simulink model "lab4_1"  (R2021b)
settings: Solver=VariableStepAuto  StartTime=0.0  StopTime=20.0  RelTol=10e-10  AbsTol=10e-10
values from neighbouring files (symbols this model uses):
  d_bar = (Ra/Kt)*tau_l    (= 3)    [lab4.m]
  thetades = pi/2    (= 1.57079632679)    [lab4.m]
  Vlim = 5    [lab4.m]
libraries: cstblocks x2
settings Model: Creator=jiayizhou  LastModifiedBy=jiayizhou

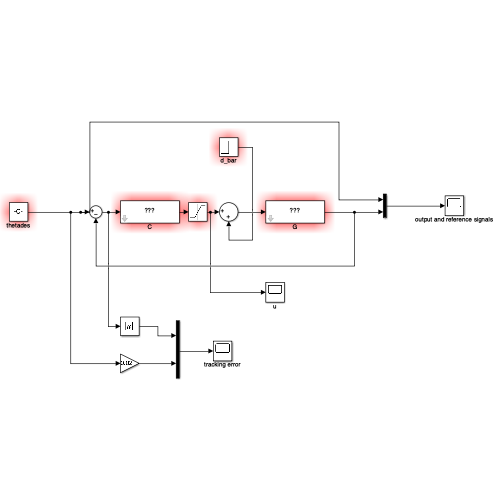
[thumbnail: Simulink's stored preview of the top-level diagram]
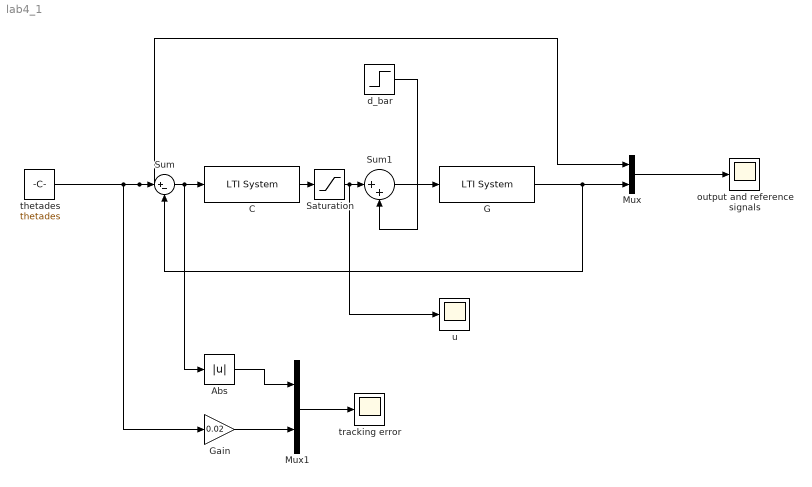
== system lab4_1 ==
  Abs : Abs
  C : cstblocks/LTI System  sys=C  IC=[]
  G : cstblocks/LTI System  sys=G  IC=[]
  Gain : Gain  Gain=0.02
  Mux : Mux  Inputs=2
  Mux1 : Mux  Inputs=2
  Saturation : Saturate  UpperLimit=Vlim  LowerLimit=-Vlim
  Sum : Sum  Inputs=|+-
  Sum1 : Sum  Inputs=|++
  d_bar : Step  Time=5  After=d_bar  SampleTime=0
  output and reference signals : Scope
  thetades : Constant  Value=thetades
  tracking error : Scope
  u : Scope
  wires:
  thetades/1 -> Gain/1, Mux/1, Sum/1
  Sum/1 -> Abs/1, C/1
  Sum1/1 -> G/1
  d_bar/1 -> Sum1/2
  Mux/1 -> output and reference signals/1
  G/1 -> Mux/2, Sum/2
  Gain/1 -> Mux1/2
  Mux1/1 -> tracking error/1
  Abs/1 -> Mux1/1
  C/1 -> Saturation/1
  Saturation/1 -> u/1, Sum1/1
